simulink model "TP4"  (R2017a)
settings: Solver=VariableStepAuto  StartTime=0.0  StopTime=10.0  RelTol=1e-3
undefined symbols (not defined in the file or in its folder): DiscIntNeverNeededParam
settings Model: Creator=rxambili  LastModifiedBy=rxambili

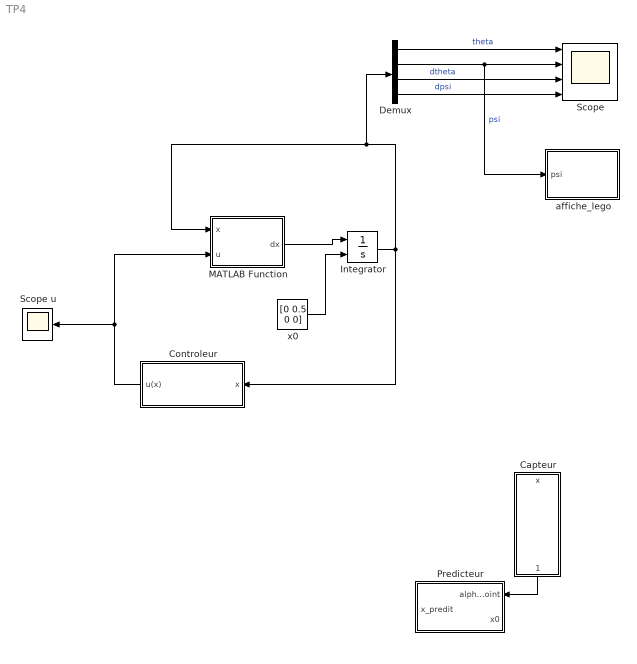
== system TP4 ==
  Capteur : Subsystem
  Controleur : Subsystem
  Demux : Demux
  Integrator : Integrator  InitialConditionSource=external
  MATLAB Function : MATLAB Function  TreatAsAtomicUnit=on
  Predicteur : Subsystem
  Scope : Scope  NumInputPorts=4
  Scope u : Scope
  "affiche_lego " : MATLAB Function  TreatAsAtomicUnit=on
  x0 : Constant  Value=[0 0.5 0 0]
  wires:
  MATLAB Function/1(dx) -> Integrator/1
  Controleur/1(u(x)) -> Scope u/1, MATLAB Function/2(u)
  x0/1 -> Integrator/2
  Demux/4 -> Scope/4  "dpsi"
  Demux/3 -> Scope/3  "dtheta"
  Demux/2 -> "affiche_lego "/1(psi), Scope/2  "psi"
  Demux/1 -> Scope/1  "theta"
  Integrator/1 -> Controleur/1(x), Demux/1, MATLAB Function/1(x)
  Capteur/1(alpha_point) -> Predicteur/1(alpha_point)

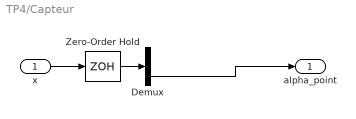
== system TP4/Capteur ==
  x : Inport
  Demux : Demux  Outputs=2
  Zero-Order Hold : ZeroOrderHold  SampleTime=-1
  alpha_point : Outport
  wires:
  x/1 -> Zero-Order Hold/1
  Demux/2 -> alpha_point/1
  Zero-Order Hold/1 -> Demux/1

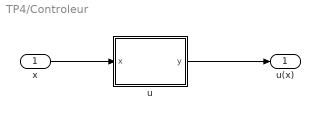
== system TP4/Controleur ==
  x : Inport
  u : MATLAB Function  TreatAsAtomicUnit=on
  u(x) : Outport
  wires:
  x/1 -> u/1(x)
  u/1(y) -> u(x)/1

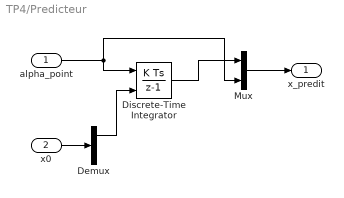
== system TP4/Predicteur ==
  alpha_point : Inport
  x0 : Inport  Port=2
  Demux : Demux  Outputs=2
  Discrete-Time Integrator : DiscreteIntegrator  InitialConditionSource=external  InitialConditionSetting=State (most efficient)  SampleTime=-1  ICPrevOutput=DiscIntNeverNeededParam  ICPrevScaledInput=DiscIntNeverNeededParam
  Mux : Mux  Inputs=2
  x_predit : Outport
  wires:
  alpha_point/1 -> Discrete-Time Integrator/1, Mux/2
  Discrete-Time Integrator/1 -> Mux/1
  Mux/1 -> x_predit/1
  x0/1 -> Demux/1
  Demux/1 -> Discrete-Time Integrator/2

== matlab function TP4/Controleur/u ==
  data: x input; y output
function y = u(x)

% Parameters
    
g = 9.81;           % gravity acceleration [m/sec^2]
m = 0.03;           % wheel weight [kg]
R = 0.04;           % wheel radius [m]
Jw = m*R^2/2;       % wheel inertia moment [kg*m^2]
M = 0.6;            % body weight [kg]
H = 0.144;          % body height [m]
L = H/2;            % distance of the center of mass from the wheel axle [m]
Jpsi = M*L^2/3;     % body pitch inertia [kgm^2]
Jm = 1e-5;          % DC motor inertia moment [kgm^2]
Rm = 6.69;          % DC motor resistance [Ohm]
Kb = 0.468;         % DC motor back EMF constant [Vsec/rad]
Kt = 0.317;         % DC motor torque constant [Nm/A]
n = 1;              % gear ratio
fm = 0.0022;        % friction coefficient between body and DC motor
fw = 0;             % friction coefficient between wheel and floor
    
ue = 0;
xe = [0; 0; 0; 0];
K = [0.0147    7.5668    0.5598    1.2965];

y = ue + K*(x-xe);

== matlab function TP4/MATLAB Function ==
  data: x input; u input; dx output
function dx = fonction(x,u)
%   Dynamic equations of motion of the segway on an axis.
%   Inputs: - x = [theta psi dtheta dpsi]
%               theta: average angle of the wheels      [rad]
%               psi: body pitch angle                   [rad]
%               dtheta: average velocity of the wheels  [rad/s]
%               dpsi: body pitch velocity               [rad/s]
%          - u: DC motor voltage (same value for both motors) [V]

    % State
    psi = x(2);
    dtheta = x(3);
    dpsi = x(4);

    % Parameters
    
    g = 9.81;           % gravity acceleration [m/sec^2]
    m = 0.03;           % wheel weight [kg]
    R = 0.04;           % wheel radius [m]
    Jw = m*R^2/2;       % wheel inertia moment [kg*m^2]
    M = 0.6;            % body weight [kg]
    H = 0.144;          % body height [m]
    L = H/2;            % distance of the center of mass from the wheel axle [m]
    Jpsi = M*L^2/3;     % body pitch inertia [kgm^2]
    Jm = 1e-5;          % DC motor inertia moment [kgm^2]
    Rm = 6.69;          % DC motor resistance [Ohm]
    Kb = 0.468;         % DC motor back EMF constant [Vsec/rad]
    Kt = 0.317;         % DC motor torque constant [Nm/A]
    n = 1;              % gear ratio
    fm = 0.0022;        % friction coefficient between body and DC motor
    fw = 0;             % friction coefficient between wheel and floor
    
    % Equations of motion
    c1 = (2*m+M)*R^2 + 2*Jw + 2*n^2*Jm;
    c2 = M*L*R*cos(psi) - 2*n^2*Jm;
    c3 = -M*L*R*dpsi^2*sin(psi);
    c4 = M*L^2 + Jpsi + 2*n^2*Jm;
    c5 = -M*g*L*sin(psi);

    alpha = Kt/Rm;
    beta = Kt*Kb/Rm + fm;

    Ftheta = alpha*(2*u) - 2*(beta+fw)*dtheta + 2*beta*dpsi;
    Fpsi = -alpha*(2*u) + 2*beta*dtheta - 2*beta*dpsi;

    ddtheta = (c4*c3 - c2*c5 + c4*Ftheta - c2*Fpsi)/(c4*c1 - c2^2);
    ddpsi = (Fpsi- c2*ddtheta - c5)/c4;
    dx = [dtheta dpsi ddtheta ddpsi]';

end

% Matrices of the linearized system
% E = [(2*m+M)*R^2+2*Jw+2*Jm   M*L*R-2*Jm; M*L*R-2*Jm   M*L^2+Jpsi+2*Jm];
% detE = det(E);

% alpha = Kt/Rm;
% beta = Kt*Kb/Rm + fm;

% A32 = -M*g*L*E(1,2)/detE;
% A42 = M*g*L*E(1,1)/detE;
% A33 = -(beta*E(2,2)+2*beta*E(1,2))/detE;
% A43 = (beta*E(1,2)+2*beta*E(1,1))/detE;
% A34 = beta*(E(2,2)+2*E(1,2))/detE;
% A44 = -beta*(E(1,2)+2*E(1,1))/detE;

% B3 = alpha*(E(2,2)/2+E(1,2))/detE;
% B4 = -alpha*(E(1,2)/2+E(1,1))/detE;

% A = [0 0 1 0;0 0 0 1; 0 A32 A33 A34; 0 A42 A43 A44];
% B = [0 0 2*B3 2*B4];

== matlab function TP4/affiche_lego  ==
  data: psi input
function affiche_lego(psi)
H = 0.144;% body height [m]
r = 0.04;
x= H*sin(psi);
y= H*cos(psi);
figure(1);
th = 0:pi/50:2*pi;
xunit = r * cos(th);
yunit = r * sin(th);
plot(xunit, yunit);
plot([x,0],[y,0]);
axis([-1.5*H 1.5*H -1.5*H 1.5*H]);
